simulink model "pacemakerA1"  (R2022a)
settings: Solver=FixedStepAuto  StartTime=0.0  StopTime=10.0  FixedStep=1e-3  RelTol=1e-3  EnableMultiTasking=on
undefined symbols (not defined in the file): D10, D11, D12, D2, D4, D5, D7, D8, D9, PTA0, PTA2, PTB23, PTB9, PTC3, PTC4, PTD0, PTD2, PTD3
libraries: frdmk64flib x9
settings Model: ExtModeTrigDuration=5  Creator=eddys  LastModifiedBy=eddys
settings OptimizationCC: EnhancedBackFolding=on  PassReuseOutputArgsAs=Individual arguments  ZeroExternalMemoryAtStartup=off  ZeroInternalMemoryAtStartup=off  MaxStackSize=64  OptimizeBlockOrder=speed  DifferentSizesBufferReuse=on  OptimizationCustomize=off  EfficientTunableParamExpr=on
settings DebuggingCC: ParameterTunabilityLossMsg=error
settings HardwareCC: ProdBitPerPointer=32  ProdBitPerSizeT=32  ProdBitPerPtrDiffT=32  ProdLargestAtomicInteger=Long  ProdLargestAtomicFloat=Double  ProdWordSize=32  ProdHWDeviceType=ARM Compatible->ARM Cortex
settings SFSimCC: MATLABDynamicMemAlloc=off
settings RTWCC: SystemTargetFile=ert.tlc  HardwareBoard=NXP FRDM-K64F  TLCOptions="-aInlineSetEventsForThisBaseRateFcn=TLC_FALSE -aSuppressMultiTaskScheduler=TLC_FALSE  -aRateBasedStepFcn=0"  TemplateMakefile=ert_default_tmf  Toolchain=GNU Tools for ARM Embedded Processors
settings CodeAppCC: ForceParamTrailComments=on  IgnoreCustomStorageClasses=off  OperatorAnnotations=on  SimulinkDataObjDesc=on  SFDataObjDesc=on  InsertBlockDesc=on
settings ERTTargetCC: ExtModeTransport=4  ExtModeMexFile=sendToCommService

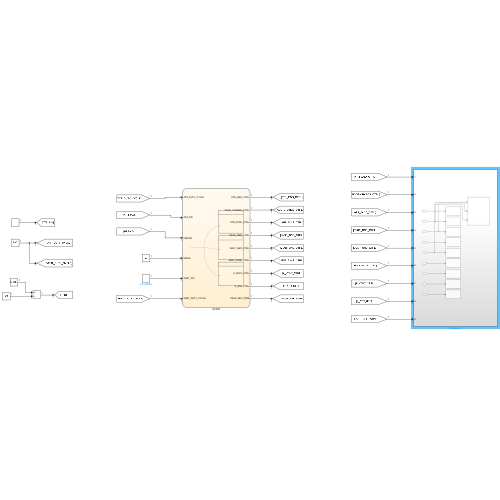
[thumbnail: Simulink's stored preview of the top-level diagram]
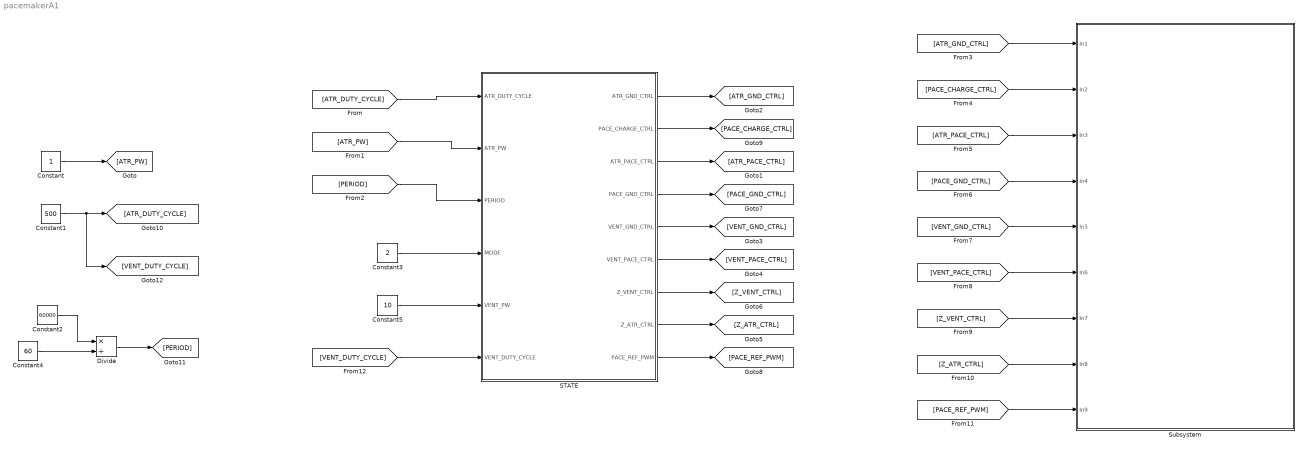
== system pacemakerA1 ==
  Constant : Constant
  Constant1 : Constant  Value=500
  Constant2 : Constant  Value=60000
  Constant3 : Constant  Value=2
  Constant4 : Constant  Value=60
  Constant5 : Constant  Value=10
  Divide : Product  Inputs=*/
  STATE : Stateflow chart  TreatAsAtomicUnit=on
  Subsystem : Subsystem
  wires:
  STATE/1(ATR_GND_CTRL) -> [ATR_GND_CTRL]
  STATE/2(PACE_CHARGE_CTRL) -> [PACE_CHARGE_CTRL]
  STATE/3(ATR_PACE_CTRL) -> [ATR_PACE_CTRL]
  STATE/4(PACE_GND_CTRL) -> [PACE_GND_CTRL]
  STATE/5(VENT_GND_CTRL) -> [VENT_GND_CTRL]
  STATE/6(VENT_PACE_CTRL) -> [VENT_PACE_CTRL]
  STATE/7(Z_VENT_CTRL) -> [Z_VENT_CTRL]
  STATE/8(Z_ATR_CTRL) -> [Z_ATR_CTRL]
  STATE/9(PACE_REF_PWM) -> [PACE_REF_PWM]
  [ATR_DUTY_CYCLE] -> STATE/1(ATR_DUTY_CYCLE)
  [ATR_PW] -> STATE/2(ATR_PW)
  [PERIOD] -> STATE/3(PERIOD)
  Constant1/1 -> [VENT_DUTY_CYCLE], [ATR_DUTY_CYCLE]
  Constant/1 -> [ATR_PW]
  Divide/1 -> [PERIOD]
  Constant4/1 -> Divide/2
  Constant2/1 -> Divide/1
  [ATR_GND_CTRL] -> Subsystem/1(In1)
  [PACE_CHARGE_CTRL] -> Subsystem/2(In2)
  [ATR_PACE_CTRL] -> Subsystem/3(In3)
  [PACE_GND_CTRL] -> Subsystem/4(In4)
  [VENT_GND_CTRL] -> Subsystem/5(In5)
  [VENT_PACE_CTRL] -> Subsystem/6(In6)
  [Z_VENT_CTRL] -> Subsystem/7(In7)
  [Z_ATR_CTRL] -> Subsystem/8(In8)
  [PACE_REF_PWM] -> Subsystem/9(In9)
  Constant3/1 -> STATE/4(MODE)
  Constant5/1 -> STATE/5(VENT_PW)
  [VENT_DUTY_CYCLE] -> STATE/6(VENT_DUTY_CYCLE)

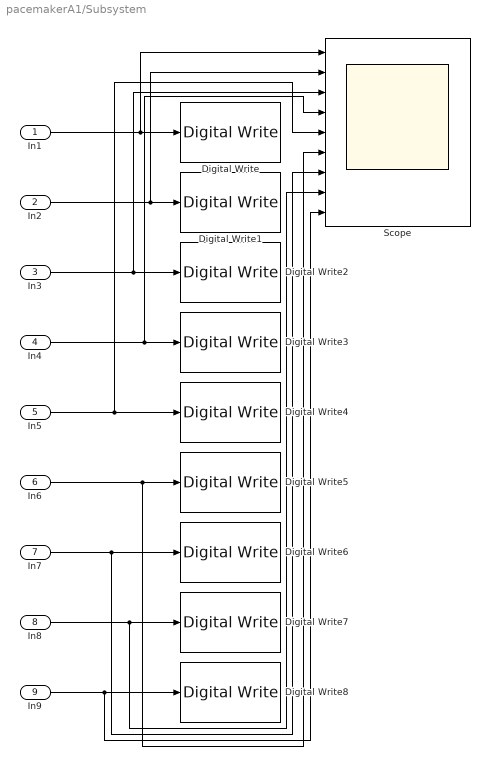
== system pacemakerA1/Subsystem ==
  In1 : Inport
  In2 : Inport  Port=2
  In3 : Inport  Port=3
  In4 : Inport  Port=4
  In5 : Inport  Port=5
  In6 : Inport  Port=6
  In7 : Inport  Port=7
  In8 : Inport  Port=8
  In9 : Inport  Port=9
  Digital Write : frdmk64flib/Digital Write  Whichpin=PTD2 (D11)
  Digital Write1 : frdmk64flib/Digital Write  Whichpin=PTB9 (D2)
  Digital Write2 : frdmk64flib/Digital Write  Whichpin=PTA0 (D8)
  Digital Write3 : frdmk64flib/Digital Write  Whichpin=PTD0 (D10)
  Digital Write4 : frdmk64flib/Digital Write  Whichpin=PTD3 (D12)
  Digital Write5 : frdmk64flib/Digital Write  Whichpin=PTC4 (D9)
  Digital Write6 : frdmk64flib/Digital Write  Whichpin=PTC3 (D7)
  Digital Write7 : frdmk64flib/Digital Write  Whichpin=PTB23 (D4)
  Digital Write8 : frdmk64flib/Digital Write  Whichpin=PTA2 (D5)
  Scope : Scope  NumInputPorts=9
  wires:
  In7/1 -> Scope/7, Digital Write6/1
  In2/1 -> Scope/2, Digital Write1/1
  In6/1 -> Scope/6, Digital Write5/1
  In4/1 -> Scope/4, Digital Write3/1
  In3/1 -> Scope/3, Digital Write2/1
  In9/1 -> Scope/9, Digital Write8/1
  In1/1 -> Scope/1, Digital Write/1
  In8/1 -> Scope/8, Digital Write7/1
  In5/1 -> Scope/5, Digital Write4/1

== stateflow chart pacemakerA1/STATE ==
  state AOO [group]
    state CharingC22
      %Capacitor charing state
      ATR_PACE_CTRL = LOW
      VENT_PACE_CTRL = LOW
      PACE_REF_PWM = ATR_DUTY_CYCLE
      PACE_CHARGE_CTRL = HIGH
      %Discharge capacitor
      PACE_GND_CTRL = HIGH
      VENT_PACE_CTRL = LOW
      Z_ATR_CTRL = LOW
      Z_VENT_CTRL = LOW
      ATR_PACE_CTRL = LOW
      ATR_GND_CTRL = LOW
      VENT_GND_CTRL = HIGH
    state AVPacing
      %step 2
      PACE_CHARGE_CTRL = LOW
      PACE_GND_CTRL = HIGH
      ATR_PACE_CTRL = HIGH
      ATR_GND_CTRL = LOW
      Z_ATR_CTRL = LOW
      Z_VENT_CTRL = LOW
      VENT_GND_CTRL = LOW
      VENT_PACE_CTRL = LOW
    CharingC22 -> AVPacing : after(PERIOD-ATR_PW, msec)
    AVPacing -> CharingC22 : after(ATR_PW, msec)
  state VOO [group]
    state CharingC23
      during:
      %Begin Charging C22 Capacitor
      ATR_PACE_CTRL = LOW
      VENT_PACE_CTRL = LOW
      PACE_REF_PWM = VENT_DUTY_CYCLE
      PACE_CHARGE_CTRL = HIGH
      %Begin Discharging C21 Blocking Capacitor
      PACE_GND_CTRL = HIGH
      VENT_PACE_CTRL = LOW
      Z_ATR_CTRL = LOW
      Z_VENT_CTRL = LOW
      ATR_PACE_CTRL = LOW
      ATR_GND_CTRL = LOW
      VENT_GND_CTRL = HIGH
    state Discharge
      during:
      %Discharge C22 into Ventricle (Vent Pacing)
      %Begin Charging Blocking Capacitor
      PACE_CHARGE_CTRL = LOW
      PACE_GND_CTRL = HIGH
      ATR_PACE_CTRL = LOW
      ATR_GND_CTRL = LOW
      Z_ATR_CTRL = LOW
      Z_VENT_CTRL = LOW
      VENT_GND_CTRL = LOW
      VENT_PACE_CTRL  = HIGH
    VOO.CharingC23 -> Discharge : after(PERIOD-VENT_PW, msec)
    Discharge -> VOO.CharingC23 : after(VENT_PW, msec)
  state TEST [group]
    state CharingC23
      %Capacitor charing state
      ATR_PACE_CTRL = LOW
      VENT_PACE_CTRL = LOW
      PACE_REF_PWM = ATR_DUTY_CYCLE
      PACE_CHARGE_CTRL = HIGH
      %Discharge capacitor
      PACE_GND_CTRL = HIGH
      VENT_PACE_CTRL = LOW
      Z_ATR_CTRL = LOW
      Z_VENT_CTRL = LOW
      ATR_PACE_CTRL = LOW
      ATR_GND_CTRL = LOW
      VENT_GND_CTRL = HIGH
    state AVPacing1
      %step 2
      PACE_CHARGE_CTRL = LOW
      PACE_GND_CTRL = HIGH
      ATR_PACE_CTRL = HIGH
      ATR_GND_CTRL = LOW
      Z_ATR_CTRL = LOW
      Z_VENT_CTRL = LOW
      VENT_GND_CTRL = LOW
      VENT_PACE_CTRL = LOW
    TEST.CharingC23 -> AVPacing1 : after(PERIOD-ATR_PW, msec)
    AVPacing1 -> TEST.CharingC23 : after(ATR_PW, msec)
  (junction 37) -> CharingC22 [order 1] : [MODE ==1]
  (junction 37) -> VOO.CharingC23 [order 2] : [MODE ==2]
  (default) -> (junction 37)
  (junction 37) -> TEST.CharingC23 [order 3]
  data: HIGH local =true; LOW local =false; ATR_GND_CTRL output; PACE_CHARGE_CTRL output; ATR_PACE_CTRL output; PACE_GND_CTRL output; VENT_GND_CTRL output; VENT_PACE_CTRL output; Z_VENT_CTRL output; Z_ATR_CTRL output; PACE_REF_PWM output; ATR_DUTY_CYCLE input; ATR_PW input; PERIOD input; MODE input; VENT_PW input; VENT_DUTY_CYCLE input
